simulink model "USV_2DOF_SS_tcurve_YAW_wPID"  (R2015b)
settings: Solver=VariableStepAuto  StartTime=0.0  StopTime=100  RelTol=1e-3
values from neighbouring files (symbols this model uses):
  breakpoints1 = data(end:-1:1,1)'    [Experimental_Impl.m]    (also in Experimental_Impl_wPlot.m; FEB02_LAKE_TEST.m; FEB14_LAKE_TEST.m; FEB28_LAKE_TEST.m)
  table_data = data(end:-1:1,2)'    [Experimental_Impl.m]    (also in Experimental_Impl_wPlot.m; FEB02_LAKE_TEST.m; FEB14_LAKE_TEST.m; FEB28_LAKE_TEST.m)
settings Model: Creator=bsb  LastModifiedBy=aschnieders22
settings ConfigComp: CovModelRefEnable=Off
settings ConfigurationSet: Description=Simscape Multibody

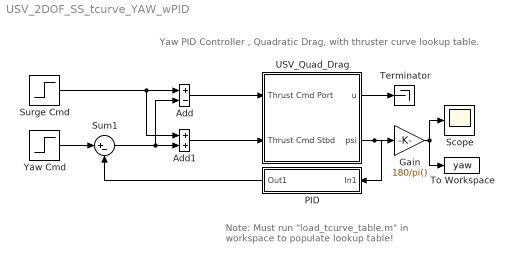
== system USV_2DOF_SS_tcurve_YAW_wPID ==
  note: Note: Must run "load_tcurve_table.m" in workspace to populate lookup table!
  note: Yaw PID Controller , Quadratic Drag, with thruster curve lookup table.
  Add : Sum  Inputs=+-
  Add1 : Sum
  Gain : Gain  Gain=180/pi()
  PID : Subsystem
  Scope : Scope
  Sum1 : Sum  Inputs=|+-
  Surge Cmd : Step  After=0  SampleTime=0
  Terminator : Terminator
  To Workspace : ToWorkspace  VariableName=yaw  SaveFormat=Timeseries  SampleTime=-1
  USV_Quad_Drag : Subsystem
  Yaw Cmd : Step  After=pi()/4  SampleTime=0
  wires:
  Surge Cmd/1 -> Add1/1, Add/1
  Add/1 -> USV_Quad_Drag/1(Thrust Cmd Port)
  Add1/1 -> USV_Quad_Drag/2(Thrust Cmd Stbd)
  USV_Quad_Drag/2(psi) -> PID/1(In1), Gain/1
  Yaw Cmd/1 -> Sum1/1
  Sum1/1 -> Add/2, Add1/2
  USV_Quad_Drag/1(u) -> Terminator/1
  PID/1(Out1) -> Sum1/2
  Gain/1 -> To Workspace/1, Scope/1

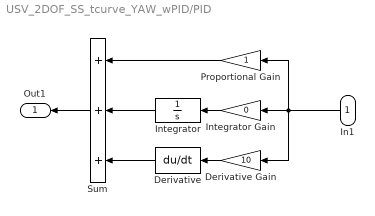
== system USV_2DOF_SS_tcurve_YAW_wPID/PID ==
  In1 : Inport
  Derivative : Derivative  CoefficientInTFapproximation=0
  Derivative Gain : Gain  Gain=10
  Integrator : TransferFcn  Denominator=[1 0]
  Integrator Gain : Gain  Gain=0
  Proportional Gain : Gain
  Sum : Sum  Inputs=+++
  Out1 : Outport
  wires:
  Derivative Gain/1 -> Derivative/1
  Integrator Gain/1 -> Integrator/1
  Proportional Gain/1 -> Sum/1
  Derivative/1 -> Sum/3
  Integrator/1 -> Sum/2
  Sum/1 -> Out1/1
  In1/1 -> Proportional Gain/1, Derivative Gain/1, Integrator Gain/1

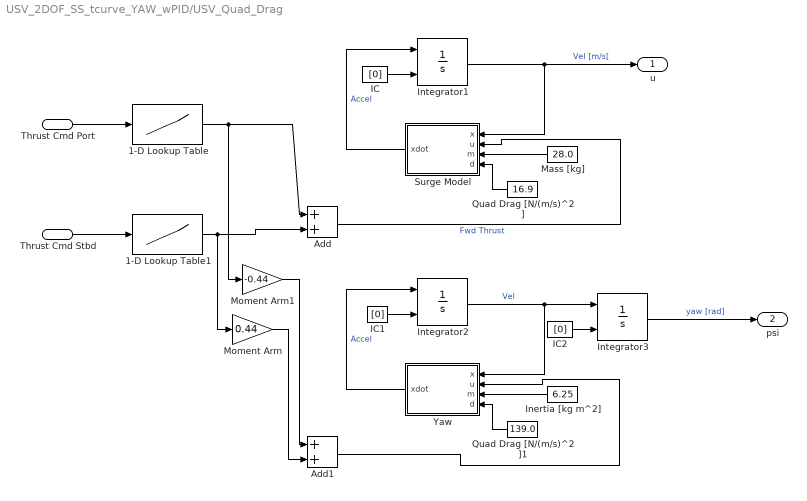
== system USV_2DOF_SS_tcurve_YAW_wPID/USV_Quad_Drag ==
  Thrust Cmd Port : Inport
  Thrust Cmd Stbd : Inport  Port=2
  1-D Lookup Table : Lookup_n-D  NumberOfTableDimensions=1  BreakpointsForDimension1=breakpoints1  Table=table_data  ExtrapMethod=Clip  UseLastTableValue=on  InternalRulePriority=Speed  RndMeth=Simplest  InputSameDT=on
  1-D Lookup Table1 : Lookup_n-D  NumberOfTableDimensions=1  BreakpointsForDimension1=breakpoints1  Table=table_data  ExtrapMethod=Clip  UseLastTableValue=on  InternalRulePriority=Speed  RndMeth=Simplest  InputSameDT=on
  Add : Sum
  Add1 : Sum
  IC : Constant  Value=[0]
  IC1 : Constant  Value=[0]
  IC2 : Constant  Value=[0]
  Inertia [kg m^2] : Constant  Value=6.25
  Integrator1 : Integrator  InitialConditionSource=external
  Integrator2 : Integrator  InitialConditionSource=external
  Integrator3 : Integrator  InitialConditionSource=external
  Mass [kg] : Constant  Value=28.0
  Moment Arm : Gain  Gain=0.44
  Moment Arm1 : Gain  Gain=-0.44
  Quad Drag [N/(m/s)^2] : Constant  Value=16.9
  Quad Drag [N/(m/s)^2]1 : Constant  Value=139.0
  Surge Model : MATLAB Function  TreatAsAtomicUnit=on
  Yaw : MATLAB Function  TreatAsAtomicUnit=on
  u : Outport
  psi : Outport  Port=2
  wires:
  IC/1 -> Integrator1/2
  Surge Model/1(xdot) -> Integrator1/1  "Accel"
  Integrator1/1 -> u/1, Surge Model/1(x)  "Vel [m/s["
  Add/1 -> Surge Model/2(u)  "Fwd Thrust"
  1-D Lookup Table/1 -> Moment Arm1/1, Add/1
  Thrust Cmd Port/1 -> 1-D Lookup Table/1
  Mass [kg]/1 -> Surge Model/3(m)
  Quad Drag [N/(m/s)^2]/1 -> Surge Model/4(d)
  1-D Lookup Table1/1 -> Moment Arm/1, Add/2
  Thrust Cmd Stbd/1 -> 1-D Lookup Table1/1
  IC1/1 -> Integrator2/2
  Yaw/1(xdot) -> Integrator2/1  "Accel"
  Integrator2/1 -> Integrator3/1, Yaw/1(x)  "Vel"
  Inertia [kg m^2]/1 -> Yaw/3(m)
  Quad Drag [N/(m/s)^2]1/1 -> Yaw/4(d)
  Integrator3/1 -> psi/1  "yaw [rad]"
  IC2/1 -> Integrator3/2
  Moment Arm1/1 -> Add1/1
  Moment Arm/1 -> Add1/2
  Add1/1 -> Yaw/2(u)

== matlab function USV_2DOF_SS_tcurve_YAW_wPID/USV_Quad_Drag/Yaw ==
  data: x input; u input; xdot output; m input; d input
function xdot = fcn(x,u,m,d)
%#codegen

% x - state of the system.  surge velocity.
% u - input. thrust force
% Model parameters
m = m; %28.0;   % Mass [kg]
d = d; %16.9;  % Quadratic drag coefficient [N/(m/s)^2]

xdot = 1/m*(-d*abs(x)*x+u);

== matlab function USV_2DOF_SS_tcurve_YAW_wPID/USV_Quad_Drag/Surge Model ==
  data: x input; u input; xdot output; m input; d input
function xdot = fcn(x,u,m,d)
%#codegen

% x - state of the system.  surge velocity.
% u - input. thrust force
% Model parameters
m = m; %28.0;   % Mass [kg]
d = d; %16.9;  % Quadratic drag coefficient [N/(m/s)^2]

xdot = 1/m*(-d*abs(x)*x+u);
